simulink model "qam64"  (R2020a)
settings: Solver=VariableStepAuto  StartTime=0.0  StopTime=10.0  RelTol=1e-3
libraries: commdigbbndam3 x2, commchan3 x1, commrandsrc3 x1
settings Model: Creator=uzend  LastModifiedBy=demid

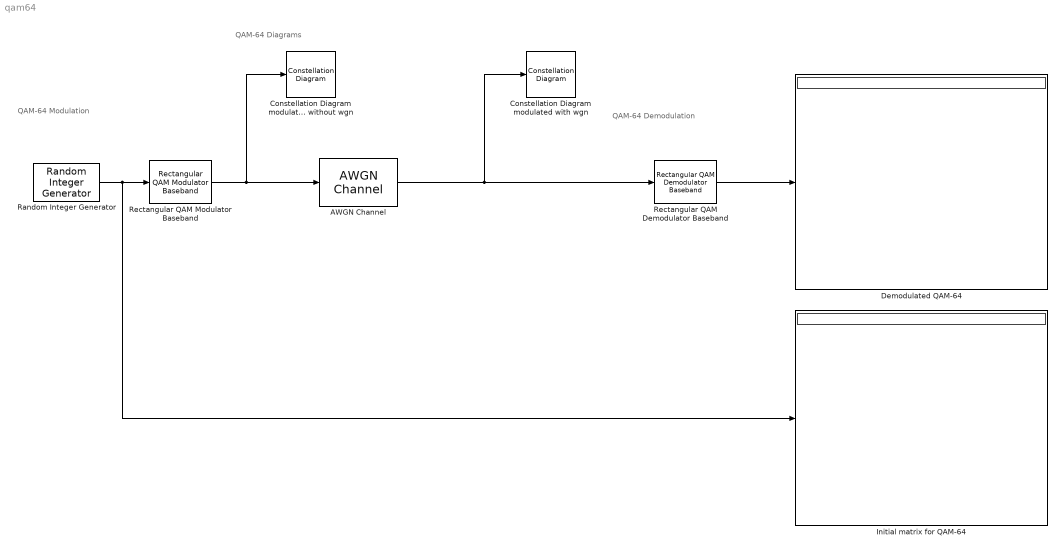
== system qam64 ==
  note: QAM-64 Demodulation
  note: QAM-64 Diagrams
  note: QAM-64 Modulation
  AWGN Channel : commchan3/AWGN Channel  InputProcessing=Columns as channels (frame based)  seed=67  noiseMode="Signal to noise ratio  (Eb/No)"  EbNodB=10  EsNodB=10  SNRdB=10  bitsPerSym=1  Ps=1  Tsym=1  variance=1
  Constellation Diagram modulated with wgn : ConstellationDiagram
  Constellation Diagram modulated without wgn : ConstellationDiagram
  Demodulated QAM-64 : Display
  Initial matrix for QAM-64 : Display
  Random Integer Generator : commrandsrc3/Random Integer Generator  SetSize=63  SeedSource=Auto  Seed=0  SampleTime=1  SamplesPerFrame=1000  OutputDataType=double  SimulateUsing=Interpreted execution
  Rectangular QAM Demodulator Baseband : commdigbbndam3/Rectangular QAM Demodulator Baseband  M=64  OutType=Integer  DecType=Hard decision  VarSource=Dialog  Variance=1  Dec=User-defined  Mapping=[0:63]  PowType=Min. distance between symbols  MinDist=2  AvgPow=1  PeakPow=1  Ph=0  outDtype1=Inherit via internal rule  outDtype2=Inherit via internal rule  derotateFactorWordLen=16  derotateFactorDataTypeStr=Inherit: Same word length as input  derotateFactorLastDataTypeStr=Inherit: Same word length as input  denormFactorWordLen=16  denormFactorDataTypeStr=Inherit: Same word length as input  denormFactorLastDataTypeStr=Inherit: Same word length as input  prodOutWordLen=32  prodOutOverflowMode=Wrap  prodOutRoundingMode=Floor  prodOutOvFlMode=off  prodOutOvFlModeLastStrValue=off  sumWordLen=32
  Rectangular QAM Modulator Baseband : commdigbbndam3/Rectangular QAM Modulator Baseband  M=64  InType=Integer  Enc=User-defined  Mapping=[0:63]  PowType=Min. distance between symbols  MinDist=2  AvgPow=1  PeakPow=1  Ph=0  outDtype=double  outWordLen=16  outUDDataType=sfix(16)  outFracLenMode=Best precision  outFracLen=15  outDataTypeStr=double  outLastDataTypeStr=double
  wires:
  Rectangular QAM Modulator Baseband/1 -> AWGN Channel/1, Constellation Diagram modulated without wgn/1
  Random Integer Generator/1 -> Rectangular QAM Modulator Baseband/1, Initial matrix for QAM-64/1
  Rectangular QAM Demodulator Baseband/1 -> Demodulated QAM-64/1
  AWGN Channel/1 -> Constellation Diagram modulated with wgn/1, Rectangular QAM Demodulator Baseband/1
